simulink model "full_Model"  (R2022b)
settings: Solver=ode15s  StartTime=0.0  StopTime=400  RelTol=1e-3
InitFcn:
  | ManipulatorSetup
  | init_quad_new_leg_raibert_strategy_v2
values from neighbouring files (symbols this model uses):
  body = 'obstacle'+string(i)    [RunModel.m]
  closeFingers = [0;0;0;0;0;0]    [ManipulatorSetup.m]
  endx = 18    [EnvironmentData.mat]
  endy = 18    [EnvironmentData.mat]
  floorl = 20    [EnvironmentData.mat]    (also in RunModel.m)
  floorw = 20    [EnvironmentData.mat]    (also in RunModel.m)
  grabObjectAngles = manipulatorAngles    [ManipulatorSetup.m]
  grabObjectAngles2 = manipulatorAngles    [ManipulatorSetup.m]
  holdFingers = [0;0;0;0;0;0]    [ManipulatorSetup.m]
  homeAngles = vertcat(configSoln.JointPosition)    [ManipulatorSetup.m]
  inverseKinematicWeights = [1 1 1 1 1 1]    [ManipulatorSetup.m]
  l1 = 0.4    [init_quad_new_leg_raibert_strategy_v2.m]
  l2 = 0.4    [init_quad_new_leg_raibert_strategy_v2.m]
  openFingers = [-20;-20;-20;-20;-20;-20]    [ManipulatorSetup.m]
  planner = plannerRRTStar(ss,stateValidator)    [RunModel.m]
  readyAngles = vertcat(configSoln.JointPosition)    [ManipulatorSetup.m]
  startx = 3    [EnvironmentData.mat]
  starty = 3    [EnvironmentData.mat]
  tar1Len = 12    [EnvironmentData.mat]    (also in RunModel.m = length(target1))
  target = [3 4.43809906251 6.0940682614 6.13591355855 7.31015448233 9.23321569187 10.9155563639 12.5209886576 14.1610706189 16.146261094 16.9318972172 17.4 ... (50 elements, 25x2)]    [EnvironmentData.mat]    (also in RunModel.m = cat(1,target1,target2))
  tarLen = 25    [EnvironmentData.mat]    (also in RunModel.m = length(target))
undefined symbols (not defined in the file or in its folder): ctrl, Extr_Data_LinkEndHole, ground, m1, m2, X, Y, Z
libraries: sm_lib x468, nesl_utility x134, slpidlib x31, robotmaniplib x6, fl_ps_legacy_lib x6, simulink x5, fl_lib x5, Contact_Forces_Lib x4, Parts_Lib x4, sharedtransform x2, dspstat3 x1
(part 15 of 16)

== system full_Model/leg_rr/upper_leg ==
  note: Geometry Only
  Cap B Left : sm_lib/Body Elements/Extruded Solid  GraphicAmbientColor=[0.15 0.15 0.15 1.0]  BasedOnType=Density  CenterOfMass=[0 0 0]  CenterOfMassUnits=m  GraphicDiffuseColor=[0.2 0.4 0.6]  ExportConvexHullGeometry=off  ExtrusionCrossSection=Extr_Data_LinkEndHole(l1*0.1,l1*0.025,0.05*l1)  ExtrusionCrossSectionUnits=m  Density=0  DensityUnits=kg/m^3  DoExposeReferenceFrame=on  GraphicEmissiveColor=[0.0 0.0 0.0 1.0]  ExportEntireGeometry=off  ExtrusionLength=l1*0.1/3  ExtrusionLengthUnits=m  ExtrusionType=General  SerializedFrames=<Frames/>  MarkerShape=Sphere  MarkerSize=10  GraphicType=FromGeometry  InertiaType=CalculateFromGeometry  Mass=1  MassUnits=kg  MomentsOfInertia=[1 1 1]  MomentsOfInertiaUnits=kg*m^2  PolygonNumSides=3  GraphicOpacity=1.0  PolygonOuterRadius=1  PolygonOuterRadiusUnits=m  ProductsOfInertia=[1 1 1]  ProductsOfInertiaUnits=kg*m^2  GraphicShininess=75  GraphicSpecularColor=[0.5 0.5 0.5 1.0]  GraphicVisPropType=SimpleVisualProperties
  Cap B Right : sm_lib/Body Elements/Extruded Solid  GraphicAmbientColor=[0.15 0.15 0.15 1.0]  BasedOnType=Density  CenterOfMass=[0 0 0]  CenterOfMassUnits=m  GraphicDiffuseColor=[0.2 0.4 0.6]  ExportConvexHullGeometry=off  ExtrusionCrossSection=Extr_Data_LinkEndHole(l1*0.1,l1*0.025,0.05*l1)  ExtrusionCrossSectionUnits=m  Density=0  DensityUnits=kg/m^3  DoExposeReferenceFrame=on  GraphicEmissiveColor=[0.0 0.0 0.0 1.0]  ExportEntireGeometry=off  ExtrusionLength=l1*0.1/3  ExtrusionLengthUnits=m  ExtrusionType=General  SerializedFrames=<Frames/>  MarkerShape=Sphere  MarkerSize=10  GraphicType=FromGeometry  InertiaType=CalculateFromGeometry  Mass=1  MassUnits=kg  MomentsOfInertia=[1 1 1]  MomentsOfInertiaUnits=kg*m^2  PolygonNumSides=3  GraphicOpacity=1.0  PolygonOuterRadius=1  PolygonOuterRadiusUnits=m  ProductsOfInertia=[1 1 1]  ProductsOfInertiaUnits=kg*m^2  GraphicShininess=75  GraphicSpecularColor=[0.5 0.5 0.5 1.0]  GraphicVisPropType=SimpleVisualProperties
  Cap F : sm_lib/Body Elements/Extruded Solid  GraphicAmbientColor=[0.15 0.15 0.15 1.0]  BasedOnType=Density  CenterOfMass=[0 0 0]  CenterOfMassUnits=m  GraphicDiffuseColor=[0.2 0.4 0.6]  ExportConvexHullGeometry=off  ExtrusionCrossSection=Extr_Data_LinkEndHole(l1*0.1,l1*0.025,0.05*l1)  ExtrusionCrossSectionUnits=m  Density=0  DensityUnits=kg/m^3  DoExposeReferenceFrame=on  GraphicEmissiveColor=[0.0 0.0 0.0 1.0]  ExportEntireGeometry=off  ExtrusionLength=l1*0.1  ExtrusionLengthUnits=m  ExtrusionType=General  SerializedFrames=<Frames/>  MarkerShape=Sphere  MarkerSize=10  GraphicType=FromGeometry  InertiaType=CalculateFromGeometry  Mass=1  MassUnits=kg  MomentsOfInertia=[1 1 1]  MomentsOfInertiaUnits=kg*m^2  PolygonNumSides=3  GraphicOpacity=1.0  PolygonOuterRadius=1  PolygonOuterRadiusUnits=m  ProductsOfInertia=[1 1 1]  ProductsOfInertiaUnits=kg*m^2  GraphicShininess=75  GraphicSpecularColor=[0.5 0.5 0.5 1.0]  GraphicVisPropType=SimpleVisualProperties
  Rigid Transform : sm_lib/Frames and Transforms/Rigid Transform  TranslationMethod=StandardAxis  TranslationStandardOffset=0.1*l1/3  TranslationLengthUnit=m  TranslationStandardAxis=+Z  TranslationCartesianOffset=[0 0 0]  TranslationROffset=0  TranslationROffsetUnits=m  TranslationZOffset=0  TranslationZOffsetUnits=m  TranslationThetaOffset=0  TranslationThetaOffsetUnits=deg  RotationMethod=StandardAxis  RotationAngleUnits=deg  RotationStandardAxis=+Z  RotationAngle=-90  RotationArbitraryAxis=[0 0 1]  FollAlignAxisA=+X  BaseAlignAxisA=+Y  FollAlignAxisB=+Y  BaseAlignAxisB=+Z  RotationSequenceAxes=FollowerAxes  RotationSequence=XYX  RotationSequenceAngles=[0 0 0]  RotationSequenceAnglesUnits=deg  RotationMatrix=[1 0 0; 0 1 0; 0 0 1]  Quaternion=[1 0 0 0]
  Transform B : sm_lib/Frames and Transforms/Rigid Transform  TranslationMethod=StandardAxis  TranslationStandardOffset=body.upper_length/2  TranslationLengthUnit=m  TranslationStandardAxis=+Y  TranslationCartesianOffset=[0 0 0]  TranslationROffset=0  TranslationROffsetUnits=m  TranslationZOffset=0  TranslationZOffsetUnits=m  TranslationThetaOffset=0  TranslationThetaOffsetUnits=deg  RotationMethod=StandardAxis  RotationAngleUnits=deg  RotationStandardAxis=+Z  RotationAngle=180  RotationArbitraryAxis=[0 0 1]  FollAlignAxisA=+X  BaseAlignAxisA=+Y  FollAlignAxisB=+Y  BaseAlignAxisB=+Z  RotationSequenceAxes=FollowerAxes  RotationSequence=XYX  RotationSequenceAngles=[0 0 0]  RotationSequenceAnglesUnits=deg  RotationMatrix=[1 0 0; 0 1 0; 0 0 1]  Quaternion=[1 0 0 0]
  Transform Cap F : sm_lib/Frames and Transforms/Rigid Transform  TranslationMethod=None  TranslationStandardOffset=0  TranslationLengthUnit=m  TranslationStandardAxis=+Z  TranslationCartesianOffset=[0 0 0]  TranslationROffset=0  TranslationROffsetUnits=m  TranslationZOffset=0  TranslationZOffsetUnits=m  TranslationThetaOffset=0  TranslationThetaOffsetUnits=deg  RotationMethod=StandardAxis  RotationAngleUnits=deg  RotationStandardAxis=+Z  RotationAngle=90  RotationArbitraryAxis=[0 0 1]  FollAlignAxisA=+X  BaseAlignAxisA=+Y  FollAlignAxisB=+Y  BaseAlignAxisB=+Z  RotationSequenceAxes=FollowerAxes  RotationSequence=XYX  RotationSequenceAngles=[0 0 0]  RotationSequenceAnglesUnits=deg  RotationMatrix=[1 0 0; 0 1 0; 0 0 1]  Quaternion=[1 0 0 0]
  Transform F : sm_lib/Frames and Transforms/Rigid Transform  TranslationMethod=None  TranslationStandardOffset=l1/2  TranslationLengthUnit=m  TranslationStandardAxis=+Y  TranslationCartesianOffset=[0 0 0]  TranslationROffset=0  TranslationROffsetUnits=m  TranslationZOffset=0  TranslationZOffsetUnits=m  TranslationThetaOffset=0  TranslationThetaOffsetUnits=deg  RotationMethod=StandardAxis  RotationAngleUnits=deg  RotationStandardAxis=+Z  RotationAngle=180  RotationArbitraryAxis=[0 0 1]  FollAlignAxisA=+X  BaseAlignAxisA=+Y  FollAlignAxisB=+Y  BaseAlignAxisB=+Z  RotationSequenceAxes=FollowerAxes  RotationSequence=XYX  RotationSequenceAngles=[0 0 0]  RotationSequenceAnglesUnits=deg  RotationMatrix=[1 0 0; 0 1 0; 0 0 1]  Quaternion=[1 0 0 0]
  Transform R : sm_lib/Frames and Transforms/Rigid Transform  TranslationMethod=StandardAxis  TranslationStandardOffset=body.upper_length/2  TranslationLengthUnit=m  TranslationStandardAxis=+Y  TranslationCartesianOffset=[0 0 0]  TranslationROffset=0  TranslationROffsetUnits=m  TranslationZOffset=0  TranslationZOffsetUnits=m  TranslationThetaOffset=0  TranslationThetaOffsetUnits=deg  RotationMethod=None  RotationAngleUnits=deg  RotationStandardAxis=+Z  RotationAngle=180  RotationArbitraryAxis=[0 0 1]  FollAlignAxisA=+X  BaseAlignAxisA=+Y  FollAlignAxisB=+Y  BaseAlignAxisB=+Z  RotationSequenceAxes=FollowerAxes  RotationSequence=XYX  RotationSequenceAngles=[0 0 0]  RotationSequenceAnglesUnits=deg  RotationMatrix=[1 0 0; 0 1 0; 0 0 1]  Quaternion=[1 0 0 0]
  "Transform Stem " : sm_lib/Frames and Transforms/Rigid Transform  TranslationMethod=StandardAxis  TranslationStandardOffset=-0.1*l1/3  TranslationLengthUnit=m  TranslationStandardAxis=+Z  TranslationCartesianOffset=[0 0 0]  TranslationROffset=0  TranslationROffsetUnits=m  TranslationZOffset=0  TranslationZOffsetUnits=m  TranslationThetaOffset=0  TranslationThetaOffsetUnits=deg  RotationMethod=StandardAxis  RotationAngleUnits=deg  RotationStandardAxis=+Z  RotationAngle=-90  RotationArbitraryAxis=[0 0 1]  FollAlignAxisA=+X  BaseAlignAxisA=+Y  FollAlignAxisB=+Y  BaseAlignAxisB=+Z  RotationSequenceAxes=FollowerAxes  RotationSequence=XYX  RotationSequenceAngles=[0 0 0]  RotationSequenceAnglesUnits=deg  RotationMatrix=[1 0 0; 0 1 0; 0 0 1]  Quaternion=[1 0 0 0]
  Upper Leg : sm_lib/Body Elements/Brick Solid  GraphicAmbientColor=[0.15 0.15 0.15 1.0]  BasedOnType=Density  BrickDimensions=[0.1*l1 body.upper_length-(l1*0.2) 0.1*l1]  BrickDimensionUnits=m  CenterOfMass=[0 0 0]  CenterOfMassUnits=m  GraphicDiffuseColor=[0.2 0.4 0.6]  Density=leg_density  DensityUnits=kg/m^3  DoExposeReferenceFrame=on  GraphicEmissiveColor=[0.0 0.0 0.0 1.0]  ExportEntireGeometry=off  SerializedFrames=<Frames><Frame><Id>Frame1</Id><Value><Name>B</Name><Origin><Source>GeometricFeature</Source><FeatureName>-y surface</FeatureName></Origin><PrimaryAxis><DefinedDirection>+Z</DefinedDirection><Source>ReferenceFrame</Source><SourceDirection>+Z</SourceDirection><FeatureName></FeatureName></PrimaryAxis><SecondaryAxis><DefinedDirection>+X</DefinedDirection><Source>ReferenceFrame</Source><SourceDirection>+X</SourceDirection><FeatureName></FeatureName></SecondaryAxis></Value></Frame><Frame><Id>Frame2</Id><Value><Name>F</Name><Origin><Source>GeometricFeature</Source><FeatureName>+y surface</FeatureName></Origin><PrimaryAxis><DefinedDirection>+Z</DefinedDirection><Source>ReferenceFrame</Source><SourceDirection>+Z</SourceDirection><FeatureName></FeatureName></PrimaryAxis><SecondaryAxis><DefinedDirection>+X</DefinedDirection><Source>ReferenceFrame</Source><SourceDirection>+X</SourceDirection><FeatureName></FeatureName></SecondaryAxis></Value></Frame></Frames>  MarkerShape=Sphere  MarkerSize=10  GraphicType=FromGeometry  InertiaType=CalculateFromGeometry  Mass=m1*l1  MassUnits=kg  MomentsOfInertia=[1 1 1]*(1/12)*m1*l1*l1^2  MomentsOfInertiaUnits=kg*m^2  GraphicOpacity=1.0  ProductsOfInertia=[1 1 1]*0  ProductsOfInertiaUnits=kg*m^2  GraphicShininess=75  GraphicSpecularColor=[0.5 0.5 0.5 1.0]  GraphicVisPropType=SimpleVisualProperties
  joint_upper : PMIOPort  Side=Right
  joint_knee : PMIOPort  Port=2  Side=Left
  connections:
  Transform Cap F/LConn1 -- Upper Leg/LConn2
  "Transform Stem "/RConn1 -- Cap B Left/RConn1
  Upper Leg/LConn1 -- "Transform Stem "/LConn1 -- Rigid Transform/LConn1
  Cap F/RConn1 -- Transform Cap F/RConn1
  Cap B Right/RConn1 -- Rigid Transform/RConn1
  Transform B/LConn1 -- Transform R/RConn1 -- Upper Leg/RConn1
  Transform B/RConn1 -- joint_upper/RConn1
  joint_knee/RConn1 -- Transform F/LConn1
  Transform F/RConn1 -- Transform R/LConn1

== system full_Model/Controller/Path follower/If Action Subsystem ==
  In1 : Inport
  Action Port : ActionPort  ActionPortLabel=if(u1 <= 0)
  Out1 : Outport
  wires:
  In1/1 -> Out1/1

== system full_Model/Controller/Path follower/If Action Subsystem1 ==
  In1 : Inport
  Action Port : ActionPort  ActionPortLabel=else
  Out1 : Outport
  wires:
  In1/1 -> Out1/1

== system full_Model/Controller/Quadruped movement Controller/Apply Target Rotation ==
  body_RotXY : Inport
  targetRotZ : Inport  Port=2
  mode : Inport  Port=3
  Constant2 : Constant  Value=0
  Constant4 : Constant
  Gain : Gain  Gain=-1
  Multiport Switch : MultiPortSwitch  Inputs=4  SaturateOnIntegerOverflow=off  InputSameDT=off
  Mux : Mux  Inputs=2
  Rotation Angles to Direction Cosine Matrix : sharedtransform/Rotation Angles to Direction Cosine Matrix  rotationOrder=XYZ  aMode=aMode
  Sum1 : Sum  Inputs=|++
  body_R : Outport
  wires:
  Mux/1 -> Rotation Angles to Direction Cosine Matrix/1
  targetRotZ/1 -> Multiport Switch/5, Gain/1
  Multiport Switch/1 -> Mux/2
  Constant2/1 -> Multiport Switch/2, Multiport Switch/3
  Sum1/1 -> Multiport Switch/1
  Constant4/1 -> Sum1/2
  Gain/1 -> Multiport Switch/4
  body_RotXY/1 -> Mux/1
  Rotation Angles to Direction Cosine Matrix/1 -> body_R/1
  mode/1 -> Sum1/1

== system full_Model/Controller/Quadruped movement Controller/Timer ==
  Compare To Constant : simulink/Logic and Bit Operations/Compare To Constant  relop=>=  const=planner.time_circle  OutDataTypeStr=boolean
  Constant4 : Constant
  Integrator : Integrator  ExternalReset=level
  Memory : Memory
  Out1 : Outport  VectorParamsAs1DForOutWhenUnconnected=off
  wires:
  Constant4/1 -> Integrator/1
  Integrator/1 -> Memory/1, Out1/1
  Compare To Constant/1 -> Integrator/2
  Memory/1 -> Compare To Constant/1

== system full_Model/Controller/Task Controller/Target Selector ==
  note: Target Position
  pos_index : Inport
  targets : Inport  Port=2
  Constant2 : Constant
  Constant3 : Constant  Value=2
  Constant4 : Constant
  Display : Display
  Display1 : Display
  If : If  IfExpression=u1 <= 0
  If Action Subsystem : Subsystem  TreatAsAtomicUnit=on
  If Action Subsystem1 : Subsystem  TreatAsAtomicUnit=on
  Memory1 : Memory
  Merge : Merge
  Mux1 : Mux  Inputs=2
  Selector : Selector  NumberOfDimensions=2  InputPortWidth=1  IndexOptions=Index vector (port),Index vector (port)  Indices=[1 3],1  OutputSizes=1,1
  Selector1 : Selector  NumberOfDimensions=2  InputPortWidth=1  IndexOptions=Index vector (port),Index vector (port)  Indices=[1 3],1  OutputSizes=1,1
  Out1 : Outport
  wires:
  If/1 -> If Action Subsystem/Action
  Constant4/1 -> If Action Subsystem/1(In1)
  Merge/1 -> Selector/2, Selector1/2
  Memory1/1 -> If Action Subsystem1/1(In1), If/1
  Selector/1 -> Mux1/1, Display/1
  Selector1/1 -> Display1/1, Mux1/2
  targets/1 -> Selector1/1, Selector/1
  If Action Subsystem1/1(Out1) -> Merge/2
  If/2 -> If Action Subsystem1/Action
  Constant2/1 -> Selector/3
  If Action Subsystem/1(Out1) -> Merge/1
  Mux1/1 -> Out1/1
  Constant3/1 -> Selector1/3
  pos_index/1 -> Memory1/1

== system full_Model/Manipulator2/Ball Tracking and Handling/Subsystem ==
  input0 : Inport
  PS Add : fl_lib/Physical Signals/Functions/PS Add
  PS Add1 : fl_lib/Physical Signals/Functions/PS Add
  PS Add2 : fl_lib/Physical Signals/Functions/PS Add
  PS Constant : fl_lib/Physical Signals/Sources/PS Constant  constant=1
  PS Product{,1..5} (6 alike) : fl_ps_legacy_lib/Legacy Physical Signals/Functions/PS Product
  PS Subtract : fl_lib/Physical Signals/Functions/PS Subtract
  Simulink-PS Converter13 : nesl_utility/Simulink-PS Converter  PhysicalDomain=network_engine_domain  SubClassName=ps_input  LeftPortType=input  RightPortType=output  PseudoPeriodic=off  Frequencies=[]  NoiseDistribution=none  NoiseParameters=[]  Unit=1  AffineConversion=off  FilteringAndDerivatives=provide  SimscapeFilterOrder=1  InputFilterTimeConstant=0.001  UdotUserProvided=0
  Conn1 : PMIOPort  Side=Left
  Conn2 : PMIOPort  Port=2  Side=Left
  Conn3 : PMIOPort  Port=3  Side=Left
  Conn4 : PMIOPort  Port=4  Side=Right
  Conn5 : PMIOPort  Port=5  Side=Left
  Conn6 : PMIOPort  Port=6  Side=Right
  Conn7 : PMIOPort  Port=7  Side=Left
  Conn8 : PMIOPort  Port=8  Side=Right
  Conn9 : PMIOPort  Port=9  Side=Left
  wires:
  input0/1 -> Simulink-PS Converter13/1
  connections:
  PS Product3/RConn1 -- PS Add1/LConn2
  PS Subtract/RConn1 -- PS Product/LConn1 -- PS Product2/LConn1 -- PS Product4/LConn1
  PS Product/RConn1 -- PS Add/LConn1
  PS Product4/RConn1 -- PS Add2/LConn1
  Conn2/RConn1 -- PS Product3/LConn2
  PS Add1/RConn1 -- Conn8/RConn1
  PS Product2/RConn1 -- PS Add1/LConn1
  PS Product5/RConn1 -- PS Add2/LConn2
  PS Subtract/LConn1 -- PS Constant/RConn1
  Simulink-PS Converter13/RConn1 -- PS Product1/LConn1 -- PS Product3/LConn1 -- PS Product5/LConn1 -- PS Subtract/LConn2
  PS Product1/RConn1 -- PS Add/LConn2
  Conn7/RConn1 -- PS Product4/LConn2
  Conn5/RConn1 -- PS Product/LConn2
  Conn9/RConn1 -- PS Product2/LConn2
  PS Add/RConn1 -- Conn4/RConn1
  Conn3/RConn1 -- PS Product5/LConn2
  Conn1/RConn1 -- PS Product1/LConn2
  PS Add2/RConn1 -- Conn6/RConn1

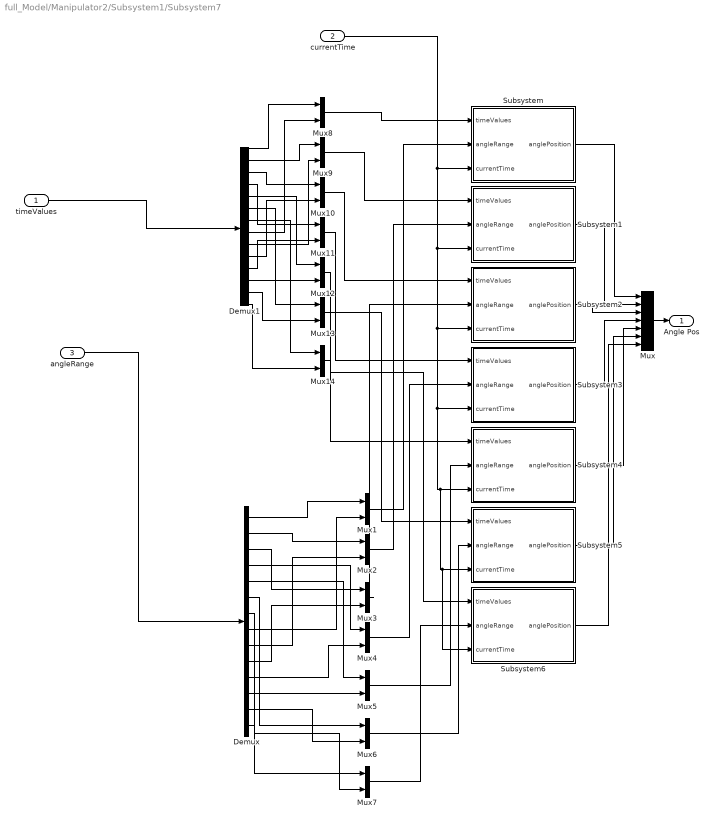
== system full_Model/Manipulator2/Subsystem1/Subsystem7 ==
  timeValues : Inport  PortDimensions=[1 14]
  currentTime : Inport  Port=2
  angleRange : Inport  Port=3
  Demux : Demux  Outputs=14
  Demux1 : Demux  Outputs=14
  Mux : Mux  Inputs=7
  Mux{1..14} (14 alike) : Mux  Inputs=2
  Subsystem : Subsystem
  Subsystem1 : Subsystem
  Subsystem2 : Subsystem
  Subsystem3 : Subsystem
  Subsystem4 : Subsystem
  Subsystem5 : Subsystem
  Subsystem6 : Subsystem
  Angle Pos : Outport
  wires:
  Subsystem3/1(anglePosition) -> Mux/4
  currentTime/1 -> Subsystem6/3(currentTime), Subsystem5/3(currentTime), Subsystem4/3(currentTime), Subsystem3/3(currentTime), Subsystem2/3(currentTime), Subsystem1/3(currentTime), Subsystem/3(currentTime)
  Subsystem2/1(anglePosition) -> Mux/3
  Subsystem/1(anglePosition) -> Mux/1
  Subsystem4/1(anglePosition) -> Mux/5
  angleRange/1 -> Demux/1
  Subsystem1/1(anglePosition) -> Mux/2
  Subsystem5/1(anglePosition) -> Mux/6
  Subsystem6/1(anglePosition) -> Mux/7
  Mux/1 -> Angle Pos/1
  Demux/1 -> Mux1/1
  Demux/8 -> Mux1/2
  Demux/2 -> Mux2/1
  Demux/9 -> Mux2/2
  Demux/3 -> Mux3/1
  Demux/10 -> Mux3/2
  Demux/4 -> Mux4/1
  Demux/11 -> Mux4/2
  Demux/5 -> Mux5/1
  Demux/12 -> Mux5/2
  Demux/6 -> Mux6/1
  Demux/13 -> Mux6/2
  Demux/7 -> Mux7/1
  Demux/14 -> Mux7/2
  Mux1/1 -> Subsystem/2(angleRange)
  Mux2/1 -> Subsystem1/2(angleRange)
  Mux3/1 -> Subsystem2/2(angleRange)
  Mux4/1 -> Subsystem3/2(angleRange)
  Mux5/1 -> Subsystem4/2(angleRange)
  Mux6/1 -> Subsystem5/2(angleRange)
  Mux7/1 -> Subsystem6/2(angleRange)
  Demux1/1 -> Mux8/1
  Demux1/2 -> Mux9/1
  Demux1/8 -> Mux8/2
  Demux1/3 -> Mux10/1
  Demux1/9 -> Mux9/2
  Demux1/10 -> Mux10/2
  Demux1/4 -> Mux11/1
  Demux1/11 -> Mux11/2
  Demux1/5 -> Mux12/1
  Demux1/12 -> Mux12/2
  Demux1/6 -> Mux13/1
  Demux1/13 -> Mux13/2
  Demux1/7 -> Mux14/1
  Demux1/14 -> Mux14/2
  Mux8/1 -> Subsystem/1(timeValues)
  Mux9/1 -> Subsystem1/1(timeValues)
  Mux10/1 -> Subsystem2/1(timeValues)
  Mux11/1 -> Subsystem3/1(timeValues)
  Mux12/1 -> Subsystem4/1(timeValues)
  Mux13/1 -> Subsystem5/1(timeValues)
  Mux14/1 -> Subsystem6/1(timeValues)
  timeValues/1 -> Demux1/1

== system full_Model/Manipulator2/inverseKinematics/If Action Subsystem ==
  T : Inport
  Action Port : ActionPort  ActionPortLabel=if(u1==1&u2==0)
  Constant7 : Constant  Value=inverseKinematicWeights
  Constant8 : Constant  Value=homeAngles
  Inverse Kinematics : robotmaniplib/Inverse Kinematics  RigidBodyTree=manipulatorModel  EndEffector=grabPositionBody  ShowInfo=off  SolverName=BFGS Gradient Projection  EnforceJointLimits=on  MaxIterations=1500  MaxTime=10  GradientTolerance=1e-7  SolutionTolerance=1e-6  StepTolerance=1e-14  ErrorChangeTolerance=1e-12  UseErrorDamping=on  DampingBias=0.0025  SimulateUsing=Interpreted execution
  objectPosition : Outport
  wires:
  Constant8/1 -> Inverse Kinematics/3
  Constant7/1 -> Inverse Kinematics/2
  T/1 -> Inverse Kinematics/1
  Inverse Kinematics/1 -> objectPosition/1

== system full_Model/Manipulator2/inverseKinematics/If Action Subsystem1 ==
  Action Port : ActionPort  ActionPortLabel=else

== system full_Model/Manipulator2/inverseKinematics/If Action Subsystem2 ==
  T : Inport
  Action Port : ActionPort  ActionPortLabel=if(u1==1&u2==0)
  Constant7 : Constant  Value=inverseKinematicWeights
  Constant8 : Constant  Value=homeAngles
  Inverse Kinematics : robotmaniplib/Inverse Kinematics  RigidBodyTree=manipulatorModel  EndEffector=grabPositionBody  ShowInfo=off  SolverName=BFGS Gradient Projection  EnforceJointLimits=on  MaxIterations=1500  MaxTime=10  GradientTolerance=1e-7  SolutionTolerance=1e-6  StepTolerance=1e-14  ErrorChangeTolerance=1e-12  UseErrorDamping=on  DampingBias=0.0025  SimulateUsing=Interpreted execution
  objectPosition : Outport
  wires:
  Constant8/1 -> Inverse Kinematics/3
  Constant7/1 -> Inverse Kinematics/2
  T/1 -> Inverse Kinematics/1
  Inverse Kinematics/1 -> objectPosition/1

== system full_Model/Manipulator2/inverseKinematics/If Action Subsystem3 ==
  Action Port : ActionPort  ActionPortLabel=else

== system full_Model/Manipulator2/inverseKinematics1/If Action Subsystem ==
  T : Inport
  Action Port : ActionPort  ActionPortLabel=if(u1==1&u2==0)
  Constant7 : Constant  Value=inverseKinematicWeights
  Constant8 : Constant  Value=homeAngles
  Inverse Kinematics : robotmaniplib/Inverse Kinematics  RigidBodyTree=manipulatorModel  EndEffector=grabPositionBody  ShowInfo=off  SolverName=BFGS Gradient Projection  EnforceJointLimits=on  MaxIterations=1500  MaxTime=10  GradientTolerance=1e-7  SolutionTolerance=1e-6  StepTolerance=1e-14  ErrorChangeTolerance=1e-12  UseErrorDamping=on  DampingBias=0.0025  SimulateUsing=Interpreted execution
  objectPosition : Outport
  wires:
  Constant8/1 -> Inverse Kinematics/3
  Constant7/1 -> Inverse Kinematics/2
  T/1 -> Inverse Kinematics/1
  Inverse Kinematics/1 -> objectPosition/1

== system full_Model/Manipulator2/inverseKinematics1/If Action Subsystem1 ==
  Action Port : ActionPort  ActionPortLabel=else

== system full_Model/Manipulator2/inverseKinematics1/If Action Subsystem2 ==
  T : Inport
  Action Port : ActionPort  ActionPortLabel=if(u1==1&u2==0)
  Constant7 : Constant  Value=inverseKinematicWeights
  Constant8 : Constant  Value=homeAngles
  Inverse Kinematics : robotmaniplib/Inverse Kinematics  RigidBodyTree=manipulatorModel  EndEffector=grabPositionBody  ShowInfo=off  SolverName=BFGS Gradient Projection  EnforceJointLimits=on  MaxIterations=1500  MaxTime=10  GradientTolerance=1e-7  SolutionTolerance=1e-6  StepTolerance=1e-14  ErrorChangeTolerance=1e-12  UseErrorDamping=on  DampingBias=0.0025  SimulateUsing=Interpreted execution
  objectPosition : Outport
  wires:
  Constant8/1 -> Inverse Kinematics/3
  Constant7/1 -> Inverse Kinematics/2
  T/1 -> Inverse Kinematics/1
  Inverse Kinematics/1 -> objectPosition/1

== system full_Model/Manipulator2/inverseKinematics1/If Action Subsystem3 ==
  Action Port : ActionPort  ActionPortLabel=else

== system full_Model/Controller/Task Controller/Target Selector/If Action Subsystem ==
  In1 : Inport
  Action Port : ActionPort  ActionPortLabel=if(u1 <= 0)
  Out1 : Outport
  wires:
  In1/1 -> Out1/1

== system full_Model/Controller/Task Controller/Target Selector/If Action Subsystem1 ==
  In1 : Inport
  Action Port : ActionPort  ActionPortLabel=else
  Out1 : Outport
  wires:
  In1/1 -> Out1/1

== system full_Model/Manipulator2/Subsystem1/Subsystem7/Subsystem ==
  timeValues : Inport
  angleRange : Inport  Port=2
  currentTime : Inport  Port=3
  1-D Lookup Table : Lookup_n-D  NumberOfTableDimensions=1  BreakpointsForDimension1Source=Input port  BreakpointsForDimension1=[-5:5]  TableSource=Input port  Table=tanh([-5:5])  InternalRulePriority=Speed  RndMeth=Simplest
      settings: InputPortMap=u0,p221,p5
  Display : Display
  anglePosition : Outport
  wires:
  timeValues/1 -> 1-D Lookup Table/3
  1-D Lookup Table/1 -> anglePosition/1
  currentTime/1 -> 1-D Lookup Table/1
  angleRange/1 -> 1-D Lookup Table/2, Display/1

== system full_Model/Manipulator2/Subsystem1/Subsystem7/Subsystem1 ==
  timeValues : Inport
  angleRange : Inport  Port=2
  currentTime : Inport  Port=3
  1-D Lookup Table : Lookup_n-D  NumberOfTableDimensions=1  BreakpointsForDimension1Source=Input port  BreakpointsForDimension1=[-5:5]  TableSource=Input port  Table=tanh([-5:5])  InternalRulePriority=Speed  RndMeth=Simplest
      settings: InputPortMap=u0,p221,p5
  anglePosition : Outport
  wires:
  timeValues/1 -> 1-D Lookup Table/3
  1-D Lookup Table/1 -> anglePosition/1
  currentTime/1 -> 1-D Lookup Table/1
  angleRange/1 -> 1-D Lookup Table/2

== system full_Model/Manipulator2/Subsystem1/Subsystem7/Subsystem2 ==
  timeValues : Inport
  angleRange : Inport  Port=2
  currentTime : Inport  Port=3
  1-D Lookup Table : Lookup_n-D  NumberOfTableDimensions=1  BreakpointsForDimension1Source=Input port  BreakpointsForDimension1=[-5:5]  TableSource=Input port  Table=tanh([-5:5])  InternalRulePriority=Speed  RndMeth=Simplest
      settings: InputPortMap=u0,p221,p5
  anglePosition : Outport
  wires:
  timeValues/1 -> 1-D Lookup Table/3
  1-D Lookup Table/1 -> anglePosition/1
  currentTime/1 -> 1-D Lookup Table/1
  angleRange/1 -> 1-D Lookup Table/2

== system full_Model/Manipulator2/Subsystem1/Subsystem7/Subsystem3 ==
  timeValues : Inport
  angleRange : Inport  Port=2
  currentTime : Inport  Port=3
  1-D Lookup Table : Lookup_n-D  NumberOfTableDimensions=1  BreakpointsForDimension1Source=Input port  BreakpointsForDimension1=[-5:5]  TableSource=Input port  Table=tanh([-5:5])  InternalRulePriority=Speed  RndMeth=Simplest
      settings: InputPortMap=u0,p221,p5
  anglePosition : Outport
  wires:
  timeValues/1 -> 1-D Lookup Table/3
  1-D Lookup Table/1 -> anglePosition/1
  currentTime/1 -> 1-D Lookup Table/1
  angleRange/1 -> 1-D Lookup Table/2

== system full_Model/Manipulator2/Subsystem1/Subsystem7/Subsystem4 ==
  timeValues : Inport
  angleRange : Inport  Port=2
  currentTime : Inport  Port=3
  1-D Lookup Table : Lookup_n-D  NumberOfTableDimensions=1  BreakpointsForDimension1Source=Input port  BreakpointsForDimension1=[-5:5]  TableSource=Input port  Table=tanh([-5:5])  InternalRulePriority=Speed  RndMeth=Simplest
      settings: InputPortMap=u0,p221,p5
  anglePosition : Outport
  wires:
  timeValues/1 -> 1-D Lookup Table/3
  1-D Lookup Table/1 -> anglePosition/1
  currentTime/1 -> 1-D Lookup Table/1
  angleRange/1 -> 1-D Lookup Table/2

== system full_Model/Manipulator2/Subsystem1/Subsystem7/Subsystem5 ==
  timeValues : Inport
  angleRange : Inport  Port=2
  currentTime : Inport  Port=3
  1-D Lookup Table : Lookup_n-D  NumberOfTableDimensions=1  BreakpointsForDimension1Source=Input port  BreakpointsForDimension1=[-5:5]  TableSource=Input port  Table=tanh([-5:5])  InternalRulePriority=Speed  RndMeth=Simplest
      settings: InputPortMap=u0,p221,p5
  anglePosition : Outport
  wires:
  timeValues/1 -> 1-D Lookup Table/3
  1-D Lookup Table/1 -> anglePosition/1
  currentTime/1 -> 1-D Lookup Table/1
  angleRange/1 -> 1-D Lookup Table/2

== system full_Model/Manipulator2/Subsystem1/Subsystem7/Subsystem6 ==
  timeValues : Inport
  angleRange : Inport  Port=2
  currentTime : Inport  Port=3
  1-D Lookup Table : Lookup_n-D  NumberOfTableDimensions=1  BreakpointsForDimension1Source=Input port  BreakpointsForDimension1=[-5:5]  TableSource=Input port  Table=tanh([-5:5])  InternalRulePriority=Speed  RndMeth=Simplest
      settings: InputPortMap=u0,p221,p5
  anglePosition : Outport
  wires:
  timeValues/1 -> 1-D Lookup Table/3
  1-D Lookup Table/1 -> anglePosition/1
  currentTime/1 -> 1-D Lookup Table/1
  angleRange/1 -> 1-D Lookup Table/2

== matlab function full_Model/Controller/Quadruped movement Controller/QuadCtrl ==
  settings: updateMethod=DISCRETE
  data: fl_ang input; tgt_ctrl_fl output; fr_ang input; rl_ang input; rr_ang input; contact_state input; body_R input; sensing_info input; tgt_ctrl_fr output; tgt_ctrl_rl output; tgt_ctrl_rr output; t input; body parameter; planner parameter; mode input; ctrl_state output; debug output; next_state input
function [tgt_ctrl_fl,tgt_ctrl_fr,tgt_ctrl_rl,tgt_ctrl_rr, ctrl_state, debug] = ...
    controller(fl_ang, fr_ang, rl_ang, rr_ang, ...
    contact_state, body_R, sensing_info, t, body, planner, mode, next_state)

%unpack sensing_info
body_vx = sensing_info(4);
body_vy = sensing_info(5);

% distance from center of mass to shoulder
fl_offset = [body.shoulder_distance;body.y_length/2+body.shoulder_size/2;0];
fr_offset = [body.shoulder_distance;-body.y_length/2-body.shoulder_size/2;0];
rl_offset = [-body.shoulder_distance;body.y_length/2+body.shoulder_size/2;0];
rr_offset = [-body.shoulder_distance;-body.y_length/2-body.shoulder_size/2;0];

%decide state and state transition helpers
persistent state;
persistent timer;
persistent timer2;
if isempty(state)
    state = 0;
end
if isempty(timer)
    timer = 0;
end
if isempty(timer2)
    timer2 = 0;
end

% init variables
           % fl fr rl rr
has_u_ctrl = [1 1 1 1];
normal_virtual_leg1 = [0;0;planner.stand_height];
normal_virtual_leg2 = [0;0;planner.stand_height];
move_fl_end_effector = normal_virtual_leg1;
move_rr_end_effector = normal_virtual_leg1;
move_fr_end_effector = normal_virtual_leg2;
move_rl_end_effector = normal_virtual_leg2;

% turning on spot mechanic
isTurning = mode == 2 || mode == 3;
%{
if isTurning
    leg_a_coef = 1; % -1/3
    leg_b_coef = 1;
else
    leg_a_coef = 1;
    leg_b_coef = 1;
end
%}
leg_a_coef = 1;
leg_b_coef = 1;

% state machine

if state == 0 % standby state
    % in this state, just do nothing, but use time to make sure that all
    % feet stands on the ground

    if contact_state(1) == 1 && contact_state(2) == 1 && contact_state(3) == 1 && contact_state(4) == 1
        %all foot on ground
        if abs(body_vx) < planner.state0_vel_thres 
            timer = timer + 1;
        else
            timer = 0;
        end
        if timer > planner.state0_trans_thres 
            state = 1;
            timer = 0;
        end
    end
elseif state == 1 % swing whole body to get a inital velocity
    timer2 = timer2 + 1;
    move_theta = planner.state0_swing_ang*sin(2*pi/planner.state0_swing_T*timer2);
    move_leg_Rx = [cos(move_theta) 0 sin(move_theta);
        0 1 0;
        -sin(move_theta) 0 cos(move_theta)];
    tgt_virtual_leg1_b = move_leg_Rx*normal_virtual_leg1;
    tgt_virtual_leg2_b = move_leg_Rx*normal_virtual_leg2;
    move_fl_end_effector = tgt_virtual_leg1_b;
    move_rr_end_effector = tgt_virtual_leg1_b;
    move_fr_end_effector = tgt_virtual_leg2_b;
    move_rl_end_effector = tgt_virtual_leg2_b;
        
    if body_vx > planner.state12_trans_speed
        timer = timer + 1;
    else
        timer = 0;
    end
    if timer > 40  %(keep a velocity larger than 0.2 for 0.1s)
        state = next_state;
        timer = 0;
        timer2 = 0;
    end

elseif state == 2 % stance virtual leg1, swing virtual leg2
    timer2 = timer2 + 1;
    if timer2 > planner.leg_swing_time %(0.5s finish movement)
        timer2 = planner.leg_swing_time;
    end
    % stance leg no u control but need to balance the body
               % fl fr rl rr
    has_u_ctrl = [0 1 1 0];
    t = timer2/planner.leg_swing_time;
%     stance_length_coeff = 0.95+0.05*(timer2/planner.leg_swing_time);
    stance_length_coeff = 0.2*t^2 - 0.2*t + 1;
    tgt_virtual_leg1_b = stance_length_coeff*normal_virtual_leg1;
    move_fl_end_effector = tgt_virtual_leg1_b;
    move_rr_end_effector = tgt_virtual_leg1_b;
    
    
    % swing leg must consider body angle 
%     move_theta = -11/180*pi*(t);
    length_coeff = 0.8*t^2-0.8*t+1;
    % move leg in x direction
    move_theta = get_move_angle(length_coeff*normal_virtual_leg2,body_vx, planner.tgt_body_vx, planner);
    
    move_leg_Rx = [cos(move_theta) 0 sin(move_theta);
        0 1 0;
        -sin(move_theta) 0 cos(move_theta)];
    move_leg_Rx2 = [cos(move_theta) 0 sin(move_theta);
        0 1 0;
        -sin(move_theta) 0 cos(move_theta)];
    tgt_virtual_leg2_a = length_coeff*move_leg_Rx2*normal_virtual_leg2;
    tgt_virtual_leg2_b = length_coeff*move_leg_Rx*normal_virtual_leg2;
    
    % move leg in y direction
    sagittal_angle = get_sagittal_angle(tgt_virtual_leg2_b,body_R, body_vy, planner);
    move_leg_Ry =[1 0 0;
                 0 cos(sagittal_angle) -sin(sagittal_angle);
                 0 sin(sagittal_angle) cos(sagittal_angle)];
    tgt_virtual_leg2_b = move_leg_Ry*tgt_virtual_leg2_b;
    tgt_virtual_leg2_a = move_leg_Ry*tgt_virtual_leg2_a;
    
    
    move_fr_end_effector = body_R'*(tgt_virtual_leg2_b+fr_offset)-fr_offset;
    if norm(move_fr_end_effector) > body.max_stretch
        move_fr_end_effector = move_fr_end_effector/norm(move_fr_end_effector)*body.max_stretch;
    end
    move_rl_end_effector = body_R'*(tgt_virtual_leg2_a+rl_offset)-rl_offset;
    if norm(move_rl_end_effector) > body.max_stretch
        move_rl_end_effector = move_rl_end_effector/norm(move_rl_end_effector)*body.max_stretch;
    end
    
    % state transition
%     if timer2 == planner.leg_swing_time
    if timer2 > 0.5*planner.leg_swing_time && contact_state(2) == 1 && contact_state(3) == 1
        timer = timer + 1;
    else
        timer = 0;
    end
    if timer > 5   % to be determined
        state = next_state;
        timer = 0;
        timer2 = 0;
    end
    
elseif state == 3 % swing virtual leg1, stance virtual leg2
    timer2 = timer2 + 1;
    if timer2 > planner.leg_swing_time %(0.5s finish movement)
        timer2 = planner.leg_swing_time;
    end
    % stance leg no u control but need to balance the body
               % fl fr rl rr
    has_u_ctrl = [1 0 0 1];
%     stance_length_coeff = 0.95+0.05*(timer2/planner.leg_swing_time);
    t = timer2/planner.leg_swing_time;
    stance_length_coeff = 0.2*t^2 - 0.2*t + 1;
    tgt_virtual_leg2_b = stance_length_coeff*normal_virtual_leg2;
    move_fr_end_effector = tgt_virtual_leg2_b;
    move_rl_end_effector = tgt_virtual_leg2_b;
    
    % swing leg must consider body angle 
    % theta is a function of forward velocity 
%     move_theta = -11/180*pi*(t);
    length_coeff = 0.8*t^2-0.8*t+1;
    move_theta = get_move_angle(length_coeff*normal_virtual_leg1,body_vx, planner.tgt_body_vx, planner);
    move_leg_Rx = [cos(move_theta*(1-2*isTurning)) 0 sin(move_theta*(1-2*isTurning));
        0 1 0;
        -sin(move_theta*(1-2*isTurning)) 0 cos(move_theta*(1-2*isTurning))];
    move_leg_Rx2 = [cos(move_theta*(1-2*isTurning)) 0 sin(move_theta*(1-2*isTurning));
        0 1 0;
        -sin(move_theta*(1-2*isTurning)) 0 cos(move_theta*(1-2*isTurning))];
    tgt_virtual_leg1_a = length_coeff*move_leg_Rx2*normal_virtual_leg1;
    tgt_virtual_leg1_b = length_coeff*move_leg_Rx*normal_virtual_leg1;
    
    % move leg in y direction
    sagittal_angle = get_sagittal_angle(tgt_virtual_leg1_b,body_R, body_vy, planner);
    move_leg_Ry =[1 0 0;
                 0 cos(sagittal_angle) -sin(sagittal_angle);
                 0 sin(sagittal_angle) cos(sagittal_angle)];
    tgt_virtual_leg1_b = move_leg_Ry*tgt_virtual_leg1_b;
    tgt_virtual_leg1_a = move_leg_Ry*tgt_virtual_leg1_a;
    
    move_fl_end_effector = body_R'*(tgt_virtual_leg1_b+fl_offset)-fl_offset;
    if norm(move_fl_end_effector) > body.max_stretch
        move_fl_end_effector = move_fl_end_effector/norm(move_fl_end_effector)*body.max_stretch;
    end
    move_rr_end_effector = body_R'*(tgt_virtual_leg1_a+rr_offset)-rr_offset;
    if norm(move_rr_end_effector) > body.max_stretch
        move_rr_end_effector = move_rr_end_effector/norm(move_rr_end_effector)*body.max_stretch;
    end
    
    % state transition
%     if timer2 == planner.leg_swing_time
    if timer2 > 0.5*planner.leg_swing_time && contact_state(1) == 1 && contact_state(4) == 1
        timer = timer + 1;
    else
        timer = 0;
    end
    if timer > 5   % to be determined
        state = next_state;
        timer = 0;
        timer2 = 0;
    end
elseif state == 4 % stabalisation
    timer2 = timer2 + 1;
    move_theta = planner.state0_swing_ang*sin(2*pi/planner.state0_swing_T*timer2);
    move_leg_Rx = [cos(move_theta) 0 sin(move_theta);
        0 1 0;
        -sin(move_theta) 0 cos(move_theta)];
    tgt_virtual_leg1_b = move_leg_Rx*normal_virtual_leg1;
    tgt_virtual_leg2_b = move_leg_Rx*normal_virtual_leg2;
    move_fl_end_effector = tgt_virtual_leg1_b;
    move_rr_end_effector = tgt_virtual_leg1_b;
    move_fr_end_effector = tgt_virtual_leg2_b;
    move_rl_end_effector = tgt_virtual_leg2_b;
        
    timer = timer + 1;
    if timer > 40  %(keep a velocity larger than 0.2 for 0.1s)
        state = next_state;
        timer = 0;
        timer2 = 0;
    end
end

%% fl to joint
[inv_s,inv_u,inv_k] = inverse_kinematics(move_fl_end_effector, body);
fl_tgt_ang_s = inv_s; 
fl_tgt_ang_u = inv_u;       
fl_tgt_ang_k = inv_k; 
tgt_ctrl_fl = [fl_tgt_ang_s;fl_tgt_ang_u;fl_tgt_ang_k;has_u_ctrl(1)];

%% fr to joint
[inv_s,inv_u,inv_k] = inverse_kinematics(move_fr_end_effector, body);
fr_tgt_ang_s = inv_s;
fr_tgt_ang_u = inv_u;
fr_tgt_ang_k = inv_k;
tgt_ctrl_fr = [fr_tgt_ang_s;fr_tgt_ang_u;fr_tgt_ang_k;has_u_ctrl(2)];

%% rl to joint
[inv_s,inv_u,inv_k] = inverse_kinematics(move_rl_end_effector, body);
rl_tgt_ang_s = inv_s;
rl_tgt_ang_u = inv_u;
rl_tgt_ang_k = inv_k;
tgt_ctrl_rl = [rl_tgt_ang_s;rl_tgt_ang_u;rl_tgt_ang_k;has_u_ctrl(3)];

%% rr to joint
[inv_s,inv_u,inv_k] = inverse_kinematics(move_rr_end_effector, body);
rr_tgt_ang_s = inv_s;
rr_tgt_ang_u = inv_u;
rr_tgt_ang_k = inv_k; 
tgt_ctrl_rr = [rr_tgt_ang_s;rr_tgt_ang_u;rr_tgt_ang_k;has_u_ctrl(4)];

ctrl_state = state;
debug = timer;

end

function move_angle = get_move_angle(virtual_leg,body_vx, tgt_body_vx, planner)

    distance = body_vx* planner.Ts/2 + planner.Kv*(tgt_body_vx-body_vx);
    
    if distance > 0.5*norm(virtual_leg)
        distance = 0.5*norm(virtual_leg);
    elseif distance < -0.5*norm(virtual_leg)
        distance = -0.5*norm(virtual_leg);
    end
    
    move_angle = asin(distance/norm(virtual_leg));
    if move_angle > 20/180*pi
        move_angle = 20/180*pi;
    elseif move_angle < -20/180*pi
        move_angle = -20/180*pi;
    end
    
end

function move_angle = get_sagittal_angle(virtual_leg,body_R, body_vy, planner)

    distance = body_vy* planner.y_Ts/2 + planner.y_Kv*(0-body_vy);  

    if distance > 0.5*norm(virtual_leg)
        distance = 0.5*norm(virtual_leg);
    elseif distance < -0.5*norm(virtual_leg)
        distance = -0.5*norm(virtual_leg);
    end
    
    move_angle = asin(distance/norm(virtual_leg));
    if move_angle > 20/180*pi
        move_angle = 20/180*pi;
    elseif move_angle < -20/180*pi
        move_angle = -20/180*pi;
    end
    
end

== stateflow chart full_Model/Controller/High Level Mode Stateflow ==
  state ResetPos
    mode=0;
    ManipTask=1;
  state Stationary
    mode=0;
    ManipTask=0;
  state Turning_Right
    mode=2;
  state Walking
    mode=1;
  state Turning_Left
    mode=3;
  Turning_Right -> ResetPos [order 2] : [resetPos==1]{pos_index=pos_index+2}
  Stationary -> ResetPos [order 2] : [resetPos==1]{pos_index=pos_index+2}
  ResetPos -> Stationary : [manipState==5]
  Walking -> ResetPos [order 4] : [resetPos==1]{pos_index=pos_index+2}
  Turning_Left -> ResetPos [order 2] : [resetPos==1]{pos_index=pos_index+2}
  (default) -> Stationary : {pos_index =2 }
  Turning_Left -> Stationary [order 1] : [delta_theta < ang_threshold]
  Turning_Right -> Stationary [order 1] : [delta_theta > -ang_threshold]
  Stationary -> Walking [order 1] : [~target_reached]
  Walking -> Stationary [order 3] : [target_reached]
      | {pos_index = pos_index + 1}
  Walking -> Turning_Right [order 2] : [delta_theta < -ang_threshold]
  Walking -> Turning_Left [order 1] : [delta_theta > ang_threshold]
  data: pos_index output =0; mode output =0; target_reached input; delta_theta input; ang_threshold local =0.2; resetPos input; ManipTask output; manipState input

== stateflow chart full_Model/Controller/Chart ==
  state PathFollowing
    resetPos=0;
  state ManipulatorTask
    resetPos=1;
  (default) -> PathFollowing
  PathFollowing -> ManipulatorTask : [pos_index==tar1Len]
  ManipulatorTask -> PathFollowing : [manipState==5]
  data: pos_index input; tar1Len input; resetPos output; manipState input

== matlab function full_Model/Manipulator2/Ball Tracking and Handling/MATLAB Function1 ==
  data: objectTransform output; x input; y input; z input; aboveObjectTransform output
function [objectTransform,aboveObjectTransform] = fcn(x,y,z)
rotTransform=[1 0 0;0 -1 0;0 0 -1];
F=rotTransform;
xline=F(1,:);
yline=F(2,:);
zline=F(3,:);
objectTransform = [ xline x;yline y;zline z+0.02;0 0 0 1];
aboveObjectTransform = [xline x;yline y;zline z+0.1;0 0 0 1];

== matlab function full_Model/Manipulator1/MATLAB Function ==
  settings: updateMethod=DISCRETE
  data: quadrupedInPosition input; errorVals input; contactForces input; state input; y output; readyAngles input; grabObjectAngles2 input; grabObjectAngles input; openFingers input; closeFingers input; holdFingers input; stateOut output; objectPosition input; aboveObjectPosition input
function [y,stateOut] = fcn(quadrupedInPosition,errorVals,contactForces,state,readyAngles,grabObjectAngles2,grabObjectAngles,openFingers,closeFingers,holdFingers,objectPosition,aboveObjectPosition)

if quadrupedInPosition == 1
    state = int16(state);

    switch state
        case 0
            y = [readyAngles;openFingers];
        case 1

            y = [aboveObjectPosition;openFingers];
        case 2
            y = [objectPosition;openFingers];
        case 3
            y = [objectPosition;closeFingers];
        case 4
            y = [aboveObjectPosition;closeFingers];
        case 5
            y = [readyAngles;closeFingers];
        otherwise
            y = zeros(13,1);
    end
    
    if state == 0 && min(errorVals) >= -0.01 && max(errorVals) <=0.01
        
        stateOut = 1;
        tic;
    elseif state == 1 && min(errorVals) >= -0.01 && max(errorVals) <=0.01 && toc >= 4
        stateOut = 2;
        tic;
    elseif state == 2 && min(errorVals) >= -0.01 && max(errorVals) <=0.01 && toc >= 0.5
        stateOut = 3;
        tic;
    elseif state == 3 && min(contactForces) >= 0.5 && toc >= 1
        toc;
        stateOut = 4;
        tic;
    elseif state == 4 && min(errorVals) >= -0.01 && max(errorVals) <=0.01 && toc >= 10
        stateOut = 5;
    elseif state == 5 && min(errorVals) >= -0.01 && max(errorVals) <=0.01
        stateOut = 5;
    else
        stateOut = double(state);
    end
else
    y = [readyAngles;openFingers];
    stateOut = 0;
end

== matlab function full_Model/Manipulator1/MATLAB Function1 ==
  data: R input; objectTransform output; x input; y input; z input; aboveObjectTransform output
function [objectTransform,aboveObjectTransform] = fcn(R,x,y,z)

objectTransform = [1 0 0 x;0 -1 0 y;0 0 -1 z+0.02;0 0 0 1];
aboveObjectTransform = [1 0 0 x;0 -1 0 y;0 0 -1 z+0.1;0 0 0 1];

== matlab function full_Model/Manipulator2/End Tracking and handling/MATLAB Function1 ==
  data: objectTransform output; x input; y input; z input; aboveObjectTransform output
function [objectTransform,aboveObjectTransform] = fcn(x,y,z)
rotTransform=[1 0 0;0 -1 0;0 0 -1];
F=rotTransform;
xline=F(1,:);
yline=F(2,:);
zline=F(3,:);
objectTransform = [ xline x;yline y;zline z+0.02;0 0 0 1];
aboveObjectTransform = [xline x;yline y;zline z+0.1;0 0 0 1];

== matlab function full_Model/Manipulator2/MATLAB Function ==
  settings: updateMethod=DISCRETE
  data: quadrupedInPosition input; errorVals input; state input; readyAngles input; openFingers input; closeFingers input; objectPosition input; aboveObjectPosition input; endPos input; aboveEndPos input; time input; y output; stateOut output; getBallPos output; getEndPos output; ballGot output
function [y,stateOut,getBallPos,getEndPos,ballGot] = fcn(quadrupedInPosition,errorVals,state,readyAngles,openFingers,closeFingers,objectPosition,aboveObjectPosition,endPos,aboveEndPos,time)

persistent startTime
if isempty(startTime)
    startTime=0;
end

threshold=0.05;
if quadrupedInPosition == 1
    state = int16(state);

    switch state
        case 0
            y = [readyAngles;openFingers];
            getBallPos=0;
            getEndPos=0;
            ballGot=0;
        case 1
            getBallPos=0;
            getEndPos=0;
            y = [aboveObjectPosition;openFingers];
            ballGot=0;
        case 2
            getBallPos=0;
            getEndPos=0;
            y = [objectPosition;openFingers];
            ballGot=0;
        case 3
            getBallPos=0;
            getEndPos=0;
            y = [objectPosition;closeFingers];
            ballGot=0;
        case 4
            getBallPos=0;
            getEndPos=0;
            y = [aboveObjectPosition;closeFingers];
            ballGot=1;
        case 5
            getBallPos=0;
            getEndPos=0;
            y = [readyAngles;closeFingers];
            ballGot=1;
        otherwise
            y = zeros(13,1);
            getBallPos=0;
            getEndPos=0;
            ballGot=0;
    end
    
    if state == 0 && min(errorVals) >= -threshold && max(errorVals) <=threshold
        getBallPos=1;
        stateOut = 1;
        startTime=time;
    elseif state == 1 && min(errorVals) >= -threshold && max(errorVals) <=threshold && (time-startTime) >= 4
        getBallPos=1;
        stateOut = 2;
        startTime=time;
    elseif state == 2  && (time-startTime) >= 4
        stateOut = 3;
        startTime=time;
    elseif state==3 && min(errorVals) >= -threshold && max(errorVals) <=threshold && (time-startTime) >= 4
        stateOut = 4;
        startTime=time;
    elseif state == 4 && min(errorVals) >= -threshold && max(errorVals) <=threshold && (time-startTime) >= 4
        stateOut = 5;
        startTime=time;
    elseif state == 5 && min(errorVals) >= -threshold && max(errorVals) <=threshold && (time-startTime)>=4
        stateOut = 5;
    else
        stateOut = double(state);
    end

elseif quadrupedInPosition == 2

    switch state
        case 5
            y = [readyAngles;closeFingers];
            getBallPos=0;
            getEndPos=0;
            ballGot=1;
        case 6
            getBallPos=0;
            getEndPos=0;
            y = [aboveEndPos;closeFingers];
            ballGot=1;
        case 7
            getBallPos=0;
            getEndPos=0;
            y = [endPos;closeFingers];
            ballGot=1;
        case 8
            getBallPos=0;
            getEndPos=0;
            y = [endPos;openFingers];
            ballGot=1;
        case 9
            getBallPos=0;
            getEndPos=0;
            y = [aboveEndPos;openFingers];
            ballGot=0;
        case 10
            getBallPos=0;
            getEndPos=0;
            y = [readyAngles;openFingers];
            ballGot=0;
        case 11
            getBallPos=0;
            getEndPos=0;
            y = [readyAngles;openFingers];
            ballGot=0;
        otherwise
            y = zeros(13,1);
            getBallPos=0;
            getEndPos=0;
            ballGot=0;
    end
    if state == 5 && min(errorVals) >= -threshold && max(errorVals) <=threshold
        stateOut = 6;
        startTime=time;
    elseif state == 6 && min(errorVals) >= -threshold && max(errorVals) <=threshold && (time-startTime) >= 4
        getEndPos=1;
        stateOut = 7;
        startTime=time;
    elseif state == 7  && (time-startTime) >= 4
        stateOut = 8;
        startTime=time;
    elseif state==8 && min(errorVals) >= -threshold && max(errorVals) <=threshold && (time-startTime) >= 5
        stateOut = 9;
        startTime=time;
    elseif state == 9 && min(errorVals) >= -threshold && max(errorVals) <=threshold && (time-startTime) >= 10
        stateOut = 10;
        startTime=time;
    elseif state == 10 && min(errorVals) >= -threshold && max(errorVals) <=threshold && (time-startTime)>=4
        stateOut = 11;
        startTime=time;
    elseif state == 11 && min(errorVals) >= -threshold && max(errorVals) <=threshold && (time-startTime)>=4
        stateOut = 11;
    else
        stateOut = double(state);
    end
else
    y = [readyAngles;openFingers];
    stateOut = 0;
    getBallPos=0;
    getEndPos=0;
    ballGot=0;
end
